simulink model "simInt"  (Simulink 7.8)
settings: Solver=ode45  StartTime=0.0  StopTime=10  RelTol=1e-3
values from neighbouring files (symbols this model uses):
  A = [0 -23.8095;0 0]    [Observador.m]    (also in P1.m; P1_pert.m; P1_pert_range.m; P1_pert_sin.m)
  B = [0;-23.8095]    [Observador.m]    (also in P1.m; P1_pert.m; P1_pert_range.m; P1_pert_sin.m)
  C = [1 0]    [Observador.m]    (also in P1.m; P1_pert.m = eye(2); P1_pert_range.m = eye(2); P1_pert_sin.m = eye(2))
  D = [0;0]    [Observador.m]    (also in P1.m; P1_pert.m; P1_pert_range.m; P1_pert_sin.m)
  K = acker(A,B,[-5+20*i -5-20*i])    [doble_integrador.m]    (also in matlab.mat = [0.749701499402 -0.42000042])
  Nu = N(3)    [Observador.m]    (also in P1.m; doble_integrador.m)
  Nx = N(1:2)    [Observador.m]    (also in P1.m; doble_integrador.m)
settings Model: Creator=student  LastModifiedBy=student

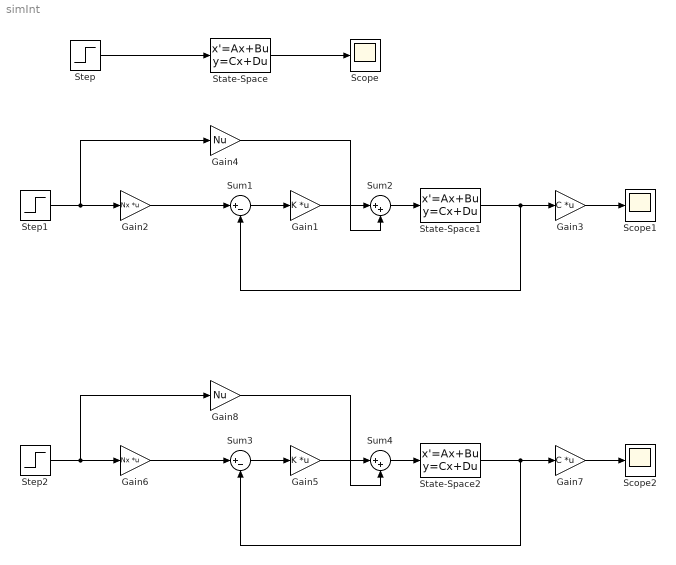
== system simInt ==
  Gain1 : Gain  Gain=K  Multiplication=Matrix(K*u)
  Gain2 : Gain  Gain=Nx  Multiplication=Matrix(K*u)
  Gain3 : Gain  Gain=C  Multiplication=Matrix(K*u)
  Gain4 : Gain  Gain=Nu
  Gain5 : Gain  Gain=K  Multiplication=Matrix(K*u)
  Gain6 : Gain  Gain=Nx  Multiplication=Matrix(K*u)
  Gain7 : Gain  Gain=C  Multiplication=Matrix(K*u)
  Gain8 : Gain  Gain=Nu
  Scope : Scope
  Scope1 : Scope
  Scope2 : Scope
      settings: SaveName=ScopeData2
  State-Space : StateSpace  A=A  B=B  C=C  D=D
  State-Space1 : StateSpace  A=A  B=B  C=eye(2)  D=D
  State-Space2 : StateSpace  A=A  B=B  C=eye(2)  D=D
  Step : Step  SampleTime=0
  Step1 : Step  SampleTime=0
  Step2 : Step  SampleTime=0
  Sum1 : Sum  Inputs=|+-
  Sum2 : Sum  Inputs=|++
  Sum3 : Sum  Inputs=|+-
  Sum4 : Sum  Inputs=|++
  wires:
  State-Space1/1 -> Gain3/1, Sum1/2
  Sum1/1 -> Gain1/1
  Step1/1 -> Gain2/1, Gain4/1
  Gain2/1 -> Sum1/1
  Gain3/1 -> Scope1/1
  Gain1/1 -> Sum2/1
  Sum2/1 -> State-Space1/1
  Gain4/1 -> Sum2/2
  State-Space/1 -> Scope/1
  Step/1 -> State-Space/1
  State-Space2/1 -> Sum3/2, Gain7/1
  Sum3/1 -> Gain5/1
  Step2/1 -> Gain8/1, Gain6/1
  Gain6/1 -> Sum3/1
  Gain7/1 -> Scope2/1
  Gain5/1 -> Sum4/1
  Sum4/1 -> State-Space2/1
  Gain8/1 -> Sum4/2
